simulink model "InvertedPendulumObserver"  (R2021b)
settings: Solver=VariableStepAuto  StartTime=0.0  StopTime=20  RelTol=1e-3
values from neighbouring files (symbols this model uses):
  A = [0 1 0 0 ... (first row only)    [linearize.m]    (also in linearize_shit.m = double(A); linearize_test.m = subs(A,omega,0); sim_lqr_control_cartpend.m; workingLinearize.m = double(A))
  B = subs(B,theta,pi)    [linearize.m]    (also in linearize_shit.m = double(B); linearize_test.m; sim_lqr_control_cartpend.m = [0; 1/M; 0; b*1/(M*L)]; workingLinearize.m = double(B))
  C = subs(C,theta,pi)    [linearize.m]    (also in linearize_shit.m = double(C); linearize_test.m = [1 0 0 0; 0 0 1 0]; workingLinearize.m = double(C))
  K = lqr(A,B,Q,R)    [sim_lqr_control_cartpend.m]    (also in workingLinearize.m)
  L = 1/2*M*xDotC^2 + 1/2*m*xDotC^2 + 1/2*m*l^2*thetaDot^2 + m*l*xDotC*thetaDot*cos(theta) + 1/2*I*thetaDot^2 + m*g*l*cos(theta)    [Calculate_lagrange.m]    (also in drawcartpend.m = 1.5; sim_cartpend.m = modelObject.L; sim_lqr_control_cartpend.m = modelObject.L; workingLinearize.m = (-place(A', C', obsPoles))')
settings Model: Creator=andre  LastModifiedBy=andre

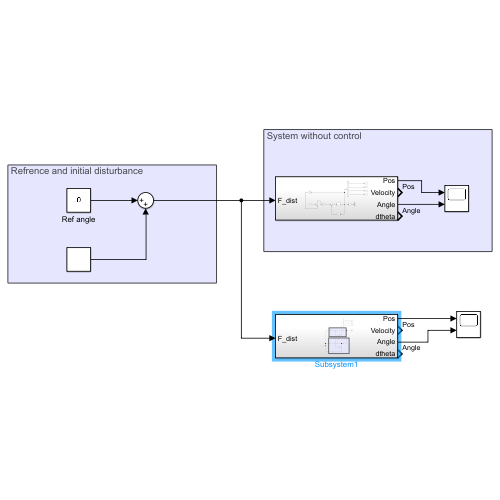
[thumbnail: Simulink's stored preview of the top-level diagram]
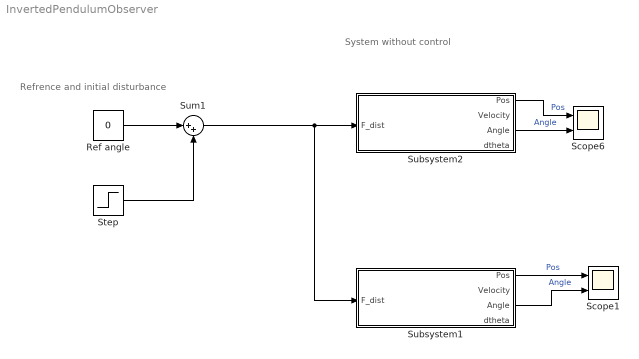
== system InvertedPendulumObserver ==
  note: Refrence and initial disturbance
  note: System without control
  Ref angle : Constant  Value=0
  Scope1 : Scope  NumInputPorts=2
  Scope6 : Scope  NumInputPorts=2
  Step : Step  Time=0.001  After=0.1  SampleTime=0
  Subsystem1 : Subsystem
  Subsystem2 : Subsystem
  Sum1 : Sum  Inputs=|++
  wires:
  Sum1/1 -> Subsystem1/1(F_dist), Subsystem2/1(F_dist)
  Step/1 -> Sum1/2
  Ref angle/1 -> Sum1/1
  Subsystem2/3(Angle) -> Scope6/2  "Angle"
  Subsystem2/1(Pos) -> Scope6/1  "Pos"
  Subsystem1/1(Pos) -> Scope1/1  "Pos"
  Subsystem1/3(Angle) -> Scope1/2  "Angle"

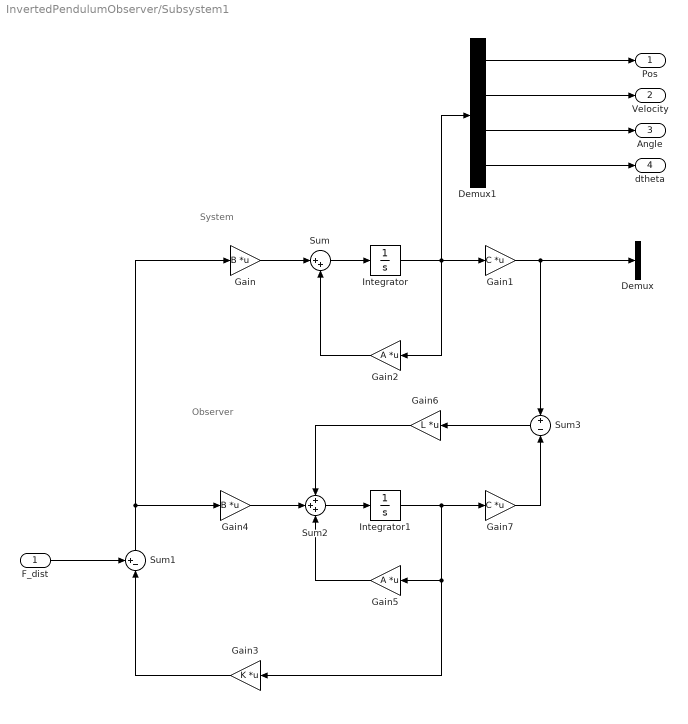
== system InvertedPendulumObserver/Subsystem1 ==
  note: System
  note: Observer
  F_dist : Inport
  Demux : Demux  Outputs=2
  Demux1 : Demux
  Gain : Gain  Gain=B  Multiplication=Matrix(K*u)
  Gain1 : Gain  Gain=C  Multiplication=Matrix(K*u)
  Gain2 : Gain  Gain=A  Multiplication=Matrix(K*u)
  Gain3 : Gain  Gain=K  Multiplication=Matrix(K*u)
  Gain4 : Gain  Gain=B  Multiplication=Matrix(K*u)
  Gain5 : Gain  Gain=A  Multiplication=Matrix(K*u)
  Gain6 : Gain  Gain=L  Multiplication=Matrix(K*u)
  Gain7 : Gain  Gain=C  Multiplication=Matrix(K*u)
  Integrator : Integrator
  Integrator1 : Integrator
  Sum : Sum  Inputs=|++
  Sum1 : Sum  Inputs=+-|
  Sum2 : Sum  Inputs=+++
  Sum3 : Sum  Inputs=+|-
  Pos : Outport
  Velocity : Outport  Port=2
  Angle : Outport  Port=3
  dtheta : Outport  Port=4
  wires:
  Demux1/3 -> Angle/1
  Integrator/1 -> Demux1/1, Gain2/1, Gain1/1
  Sum/1 -> Integrator/1
  Demux1/1 -> Pos/1
  Demux1/2 -> Velocity/1
  Gain1/1 -> Demux/1, Sum3/1
  Demux1/4 -> dtheta/1
  Gain2/1 -> Sum/2
  Gain/1 -> Sum/1
  F_dist/1 -> Sum1/1
  Gain3/1 -> Sum1/2
  Sum1/1 -> Gain/1, Gain4/1
  Gain4/1 -> Sum2/2
  Gain6/1 -> Sum2/1
  Gain5/1 -> Sum2/3
  Sum2/1 -> Integrator1/1
  Integrator1/1 -> Gain7/1, Gain5/1, Gain3/1
  Sum3/1 -> Gain6/1
  Gain7/1 -> Sum3/2

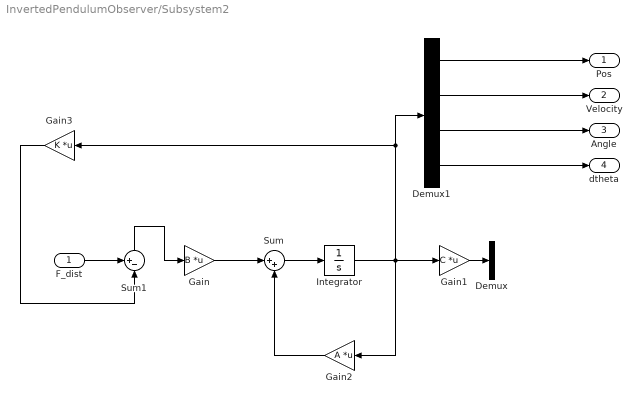
== system InvertedPendulumObserver/Subsystem2 ==
  F_dist : Inport
  Demux : Demux  Outputs=2
  Demux1 : Demux
  Gain : Gain  Gain=B  Multiplication=Matrix(K*u)
  Gain1 : Gain  Gain=C  Multiplication=Matrix(K*u)
  Gain2 : Gain  Gain=A  Multiplication=Matrix(K*u)
  Gain3 : Gain  Gain=K  Multiplication=Matrix(K*u)
  Integrator : Integrator
  Sum : Sum  Inputs=|++
  Sum1 : Sum  Inputs=+-|
  Pos : Outport
  Velocity : Outport  Port=2
  Angle : Outport  Port=3
  dtheta : Outport  Port=4
  wires:
  Demux1/3 -> Angle/1
  Integrator/1 -> Gain3/1, Demux1/1, Gain2/1, Gain1/1
  Sum/1 -> Integrator/1
  Demux1/1 -> Pos/1
  Demux1/2 -> Velocity/1
  Gain1/1 -> Demux/1
  Demux1/4 -> dtheta/1
  Gain2/1 -> Sum/2
  Gain/1 -> Sum/1
  Gain3/1 -> Sum1/2
  F_dist/1 -> Sum1/1
  Sum1/1 -> Gain/1
